simulink model "fifio_with_D2"  (R2024a)
settings: Solver=VariableStepAuto  StartTime=0.0  StopTime=0.5  RelTol=1e-3
values from neighbouring files (symbols this model uses):
  enable_FIFO_out = Ts*9009    (= 0.0675681756818)    [new_generation_coeff.m]
  Ts = 1/Fs    (= 7.50007500075e-06)    [new_generation_coeff.m]    (also in simon_test.m; simple_fft_test.m = 1/F; testPSD_c2d.m; testPSD_simulink.m)
undefined symbols (not defined in the file or in its folder): magnitude
libraries: hdlsllib x127, dsphdlxfrm2 x1
settings Model: DataTypeOverride=Off  Creator=Simon  LastModifiedBy=Simon
settings OptimizationCC: BlockReduction=off  ConditionallyExecuteInputs=off  DefaultParameterBehavior=Inlined  InheritOutputTypeSmallerThanSingle=on
settings DebuggingCC: AlgebraicLoopMsg=error  SingleTaskRateTransMsg=error  UnconnectedInputMsg=warning  UnconnectedOutputMsg=warning  UnconnectedLineMsg=warning
settings HardwareCC: ProdBitPerPointer=32  ProdBitPerSizeT=32  ProdBitPerPtrDiffT=32  ProdLargestAtomicFloat=None  ProdIntDivRoundTo=Undefined  ProdEndianess=Unspecified  ProdWordSize=32  ProdHWDeviceType=ASIC/FPGA->ASIC/FPGA  TargetBitPerPointer=64  TargetBitPerSizeT=64  TargetBitPerPtrDiffT=64  TargetLongLongMode=on  TargetIntDivRoundTo=Zero  TargetEndianess=LittleEndian  TargetWordSize=64  TargetHWDeviceType=Custom Processor->MATLAB Host Computer  ProdEqTarget=off

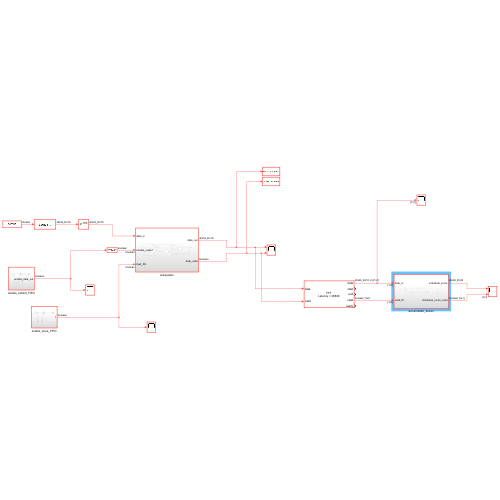
[thumbnail: Simulink's stored preview of the top-level diagram]
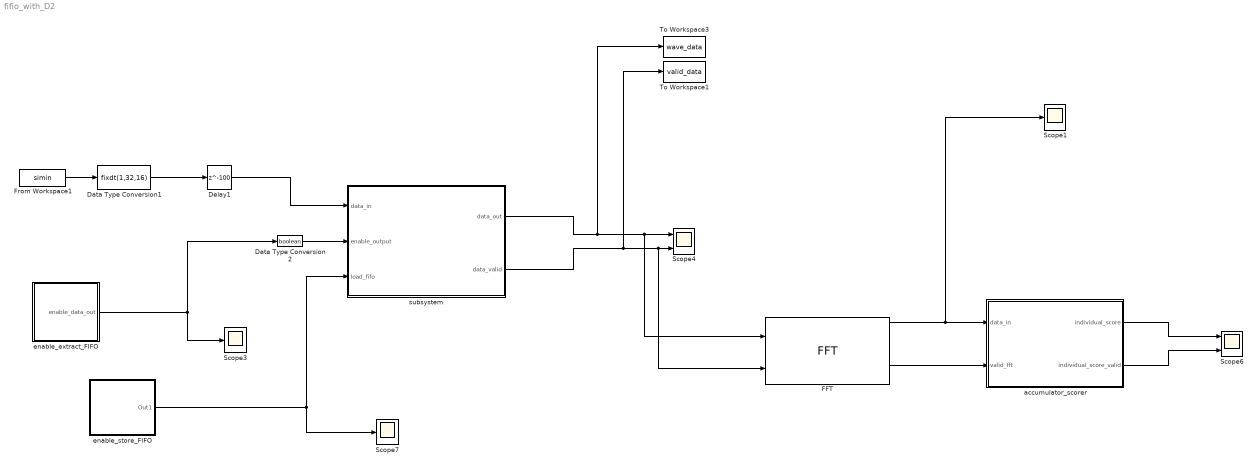
== system fifio_with_D2 ==
  Data Type Conversion1 : DataTypeConversion  OutDataTypeStr=fixdt(1,32,16)  SaturateOnIntegerOverflow=off  RndMeth=Floor
  Data Type Conversion2 : DataTypeConversion  OutDataTypeStr=boolean  SaturateOnIntegerOverflow=off  RndMeth=Floor
  Delay1 : Delay  DelayLength=100  InitialCondition=0  SampleTime=Ts
  FFT : dsphdlxfrm2/FFT  Architecture=Burst Radix 2  FFTLengthSource=Property  FFTLength=4096  FFTLengthMax=1024  ComplexMultiplication=Use 4 multipliers and 2 adders  BitReversedOutput=off  BitReversedInput=off  Normalize=off  SimulateUsing=Code generation  RoundingMethod=Floor  ResetInputPort=off  StartOutputPort=on  EndOutputPort=on
  From Workspace1 : FromWorkspace  VariableName=simin  SampleTime=Ts
  Scope1 : Scope
  Scope3 : Scope
  Scope4 : Scope  NumInputPorts=2
  Scope6 : Scope  NumInputPorts=2
  Scope7 : Scope
  To Workspace1 : ToWorkspace  VariableName=valid_data  SampleTime=Ts
  To Workspace3 : ToWorkspace  VariableName=wave_data  SampleTime=Ts
  accumulator_scorer : Subsystem
  enable_extract_FIFO : Subsystem
  enable_store_FIFO : Subsystem
  subsystem : Subsystem
  wires:
  enable_store_FIFO/1(Out1) -> subsystem/3(load_fifo), Scope7/1
  FFT/1 -> Scope1/1, accumulator_scorer/1(data_in)
  enable_extract_FIFO/1(enable_data_out) -> Data Type Conversion2/1, Scope3/1
  Data Type Conversion2/1 -> subsystem/2(enable_output)
  FFT/4 -> accumulator_scorer/2(valid_fft)
  accumulator_scorer/1(individual_score) -> Scope6/1
  Data Type Conversion1/1 -> Delay1/1
  subsystem/2(data_valid) -> FFT/2, Scope4/2, To Workspace1/1
  accumulator_scorer/2(individual_score_valid) -> Scope6/2
  From Workspace1/1 -> Data Type Conversion1/1
  Delay1/1 -> subsystem/1(data_in)
  subsystem/1(data_out) -> To Workspace3/1, FFT/1, Scope4/1

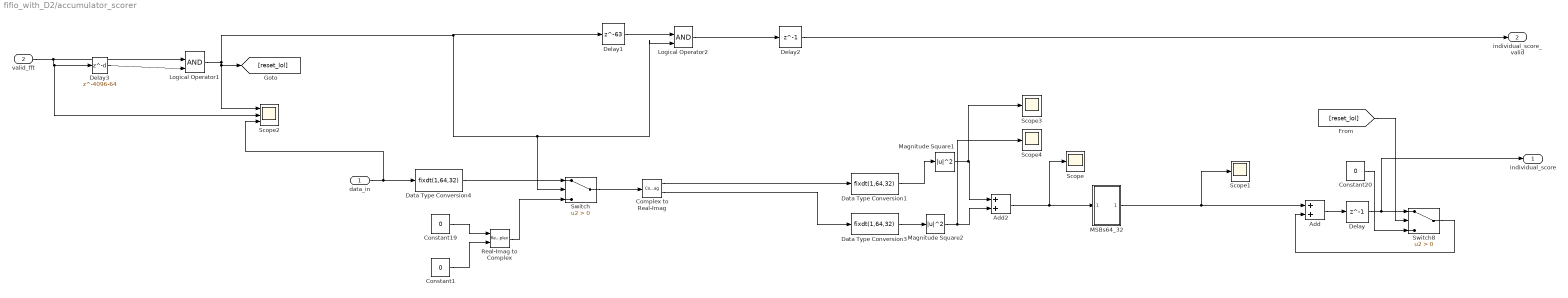
== system fifio_with_D2/accumulator_scorer ==
  data_in : Inport
  valid_fft : Inport  Port=2
  Add : Sum  OutDataTypeStr=fixdt(1,64,32)  AccumDataTypeStr=fixdt(1,64,32)
  Add2 : Sum  OutDataTypeStr=fixdt(1,64,32)  AccumDataTypeStr=fixdt(1,64,32)
  Complex to Real-Imag : ComplexToRealImag
  Constant1 : Constant  Value=0  OutDataTypeStr=fixdt(1,64,32)  SampleTime=Ts
  Constant19 : Constant  Value=0  OutDataTypeStr=fixdt(1,64,32)  SampleTime=Ts
  Constant20 : Constant  Value=0  OutDataTypeStr=fixdt(1,64,32)  SampleTime=Ts
  Data Type Conversion1 : DataTypeConversion  OutDataTypeStr=fixdt(1,64,32)  SaturateOnIntegerOverflow=off  RndMeth=Floor
  Data Type Conversion3 : DataTypeConversion  OutDataTypeStr=fixdt(1,64,32)  SaturateOnIntegerOverflow=off  RndMeth=Floor
  Data Type Conversion4 : DataTypeConversion  OutDataTypeStr=fixdt(1,64,32)  SaturateOnIntegerOverflow=off  RndMeth=Floor
  Delay : Delay  DelayLength=1  InitialCondition=0  SampleTime=Ts
  Delay1 : Delay  DelayLength=63  InitialCondition=0
  Delay2 : Delay  DelayLength=1  InitialCondition=0
  Delay3 : Delay  DelayLength=4096-64  InitialCondition=0
  Logical Operator1 : Logic  IconShape=distinctive  AllPortsSameDT=off  OutDataTypeStr=boolean
  Logical Operator2 : Logic  IconShape=distinctive  AllPortsSameDT=off  OutDataTypeStr=boolean
  MSBs64_32 : Subsystem
  Magnitude Square1 : Math  Operator=magnitude^2  SignedPower=on  OutputSignalType=real  OutDataTypeStr=fixdt(1,64,32)  RndMeth=Zero
  Magnitude Square2 : Math  Operator=magnitude^2  SignedPower=on  OutputSignalType=real  OutDataTypeStr=fixdt(1,64,32)  RndMeth=Zero
  Real-Imag to Complex : RealImagToComplex
  Scope{,1,3..4} (4 alike) : Scope
  Scope2 : Scope  NumInputPorts=3
  Switch : Switch  Criteria=u2 > Threshold  OutDataTypeStr=fixdt(1,64,32)  SaturateOnIntegerOverflow=off  InputSameDT=off
  Switch8 : Switch  Criteria=u2 > Threshold  OutDataTypeStr=fixdt(1,64,32)  SaturateOnIntegerOverflow=off  InputSameDT=off
  individual_score : Outport
  individual_score_valid : Outport  Port=2
  wires:
  Real-Imag to Complex/1 -> Switch/3
  Switch8/1 -> Add/2
  Switch/1 -> Complex to Real-Imag/1
  Delay/1 -> individual_score/1, Switch8/1
  [reset_lol] -> Switch8/2
  Add/1 -> Delay/1
  Constant20/1 -> Switch8/3
  data_in/1 -> Scope2/3, Data Type Conversion4/1
  Data Type Conversion3/1 -> Magnitude Square2/1
  Data Type Conversion1/1 -> Magnitude Square1/1
  Magnitude Square1/1 -> Scope3/1, Add2/1
  Complex to Real-Imag/1 -> Data Type Conversion1/1
  Add2/1 -> MSBs64_32/1(In1), Scope/1
  Complex to Real-Imag/2 -> Data Type Conversion3/1
  Magnitude Square2/1 -> Scope4/1, Add2/2
  Logical Operator1/1 -> Scope2/1, [reset_lol], Logical Operator2/2, Switch/2, Delay1/1
  Data Type Conversion4/1 -> Switch/1
  Constant1/1 -> Real-Imag to Complex/2
  Constant19/1 -> Real-Imag to Complex/1
  MSBs64_32/1(out) -> Scope1/1, Add/1
  Delay1/1 -> Logical Operator2/1
  Logical Operator2/1 -> Delay2/1
  Delay2/1 -> individual_score_valid/1
  valid_fft/1 -> Scope2/2, Delay3/1, Logical Operator1/1
  Delay3/1 -> Logical Operator1/2

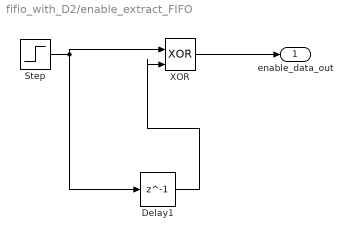
== system fifio_with_D2/enable_extract_FIFO ==
  Delay1 : Delay  DelayLength=1  InitialCondition=0  SampleTime=Ts
  Step : Step  Time=enable_FIFO_out  SampleTime=Ts
  XOR : Logic  Operator=XOR  IconShape=distinctive  AllPortsSameDT=off  OutDataTypeStr=boolean
  enable_data_out : Outport  OutDataTypeStr=boolean
  wires:
  Delay1/1 -> XOR/2
  Step/1 -> Delay1/1, XOR/1
  XOR/1 -> enable_data_out/1

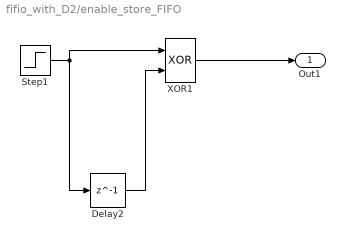
== system fifio_with_D2/enable_store_FIFO ==
  Delay2 : Delay  DelayLength=1  InitialCondition=0  SampleTime=Ts
  Step1 : Step  Time=Ts*100  SampleTime=Ts
  XOR1 : Logic  Operator=XOR  IconShape=distinctive  AllPortsSameDT=off  OutDataTypeStr=boolean
  Out1 : Outport  OutDataTypeStr=boolean
  wires:
  XOR1/1 -> Out1/1
  Step1/1 -> Delay2/1, XOR1/1
  Delay2/1 -> XOR1/2

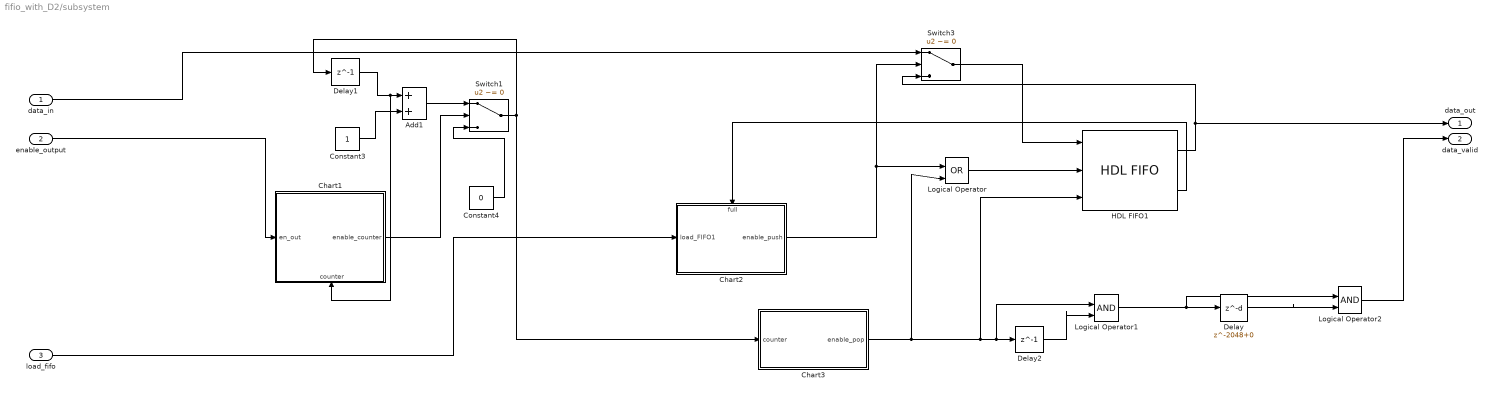
== system fifio_with_D2/subsystem ==
  data_in : Inport
  enable_output : Inport  Port=2  OutDataTypeStr=boolean
  load_fifo : Inport  Port=3  OutDataTypeStr=boolean
  Add1 : Sum  OutDataTypeStr=fixdt(0,13,0)
  Chart1 : Stateflow chart  TreatAsAtomicUnit=on
      settings: PortSchema="{\"entries\":[{\"content\":{\"sides\":[{\"content\":{\"connectorIds\":[\"In2\"]},\"type\":\"ConnectorPlacement.EquallySpacedRectSide\",\"uuid\":\"9d6f18ef-7bce-40b0-94a2-758e33355834\"},{\"content\":{\"connectorIds\":[\"Out1\"],\"side\":\"RIGHT\"},\"type\":\"ConnectorPlacement.EquallySpacedRectSide\",\"uuid\":\"7bab70ba-8111-4145-9c29-33f98ce79820\"},{\"content\":{\"side\":\"TOP\"},\"type\":\"ConnectorPlacement.EquallySpacedRectSide\",\"uuid\":\"d3288235-814f-4c71-bec2-04d07c53d63c\"},{\"content\":{\"connectorIds\":[\"In1\"],\"side\":\"BOTTOM\"},\"type\":\"ConnectorPlacement.EquallySpacedRectSide\",\"uuid\":\"018953e5-55f4-4114-8f5d-132f3f7565f7\"}]},\"type\":\"ConnectorPlacement.EquallySpacedConnector\",\"uuid\":\"70011da9-c6ae-4e69-953f-1d8cbe8c7c12\"}],\"packageUris\":[\"http://schema.mathworks.com/mf0/Connector/R2020b\"],\"version\":\"1.0\"}"
  Chart2 : Stateflow chart  TreatAsAtomicUnit=on
      settings: PortSchema="{\"entries\":[{\"content\":{\"sides\":[{\"content\":{\"connectorIds\":[\"In1\"]},\"type\":\"ConnectorPlacement.EquallySpacedRectSide\",\"uuid\":\"9d6f18ef-7bce-40b0-94a2-758e33355834\"},{\"content\":{\"connectorIds\":[\"Out1\"],\"side\":\"RIGHT\"},\"type\":\"ConnectorPlacement.EquallySpacedRectSide\",\"uuid\":\"7bab70ba-8111-4145-9c29-33f98ce79820\"},{\"content\":{\"connectorIds\":[\"In2\"],\"side\":\"TOP\"},\"type\":\"ConnectorPlacement.EquallySpacedRectSide\",\"uuid\":\"d3288235-814f-4c71-bec2-04d07c53d63c\"}]},\"type\":\"ConnectorPlacement.EquallySpacedConnector\",\"uuid\":\"70011da9-c6ae-4e69-953f-1d8cbe8c7c12\"}],\"packageUris\":[\"http://schema.mathworks.com/mf0/Connector/R2020b\"],\"version\":\"1.0\"}"
  Chart3 : Stateflow chart  TreatAsAtomicUnit=on
  Constant3 : Constant  OutDataTypeStr=fixdt(0,12,0)  SampleTime=Ts
  Constant4 : Constant  Value=0  OutDataTypeStr=fixdt(1,13,0)  SampleTime=Ts
  Delay : Delay  DelayLength=2048+0  InitialCondition=0
  Delay1 : Delay  DelayLength=1  InitialCondition=0  SampleTime=Ts
  Delay2 : Delay  DelayLength=1  InitialCondition=0  SampleTime=Ts
  HDL FIFO1 : hdlsllib/HDL RAMs/HDL FIFO  fifo_size=4096+2048+1  mode=Classic  ratio=1  push_msg=Warning  pop_msg=Warning  show_empty=off  show_full=on  show_num=off  LabelModeActiveChoice_Mode=Classic  rst_port=off
  Logical Operator : Logic  Operator=OR  IconShape=distinctive  AllPortsSameDT=off  OutDataTypeStr=boolean
  Logical Operator1 : Logic  IconShape=distinctive  AllPortsSameDT=off  OutDataTypeStr=boolean
  Logical Operator2 : Logic  IconShape=distinctive  AllPortsSameDT=off  OutDataTypeStr=boolean
  Switch1 : Switch  Criteria=u2 ~= 0  OutDataTypeStr=fixdt(0,13,0)  SaturateOnIntegerOverflow=off  InputSameDT=off
  Switch3 : Switch  Criteria=u2 ~= 0  SaturateOnIntegerOverflow=off  InputSameDT=off  OutDataTypeStr=Inherit: Same as first input
  data_out : Outport
  data_valid : Outport  Port=2
  wires:
  Delay1/1 -> Chart1/1(counter), Add1/1
  Logical Operator/1 -> HDL FIFO1/2
  HDL FIFO1/1 -> data_out/1, Switch3/3
  Switch1/1 -> Chart3/1(counter), Delay1/1
  Delay2/1 -> Logical Operator1/2
  enable_output/1 -> Chart1/2(en_out)
  Add1/1 -> Switch1/1
  Constant3/1 -> Add1/2
  HDL FIFO1/2 -> Chart2/2(full)
  Switch3/1 -> HDL FIFO1/1
  Constant4/1 -> Switch1/3
  Logical Operator1/1 -> Logical Operator2/1, Delay/1
  load_fifo/1 -> Chart2/1(load_FIFO1)
  data_in/1 -> Switch3/1
  Chart3/1(enable_pop) -> HDL FIFO1/3, Logical Operator1/1, Delay2/1, Logical Operator/2
  Chart1/1(enable_counter) -> Switch1/2
  Chart2/1(enable_push) -> Switch3/2, Logical Operator/1
  Delay/1 -> Logical Operator2/2
  Logical Operator2/1 -> data_valid/1

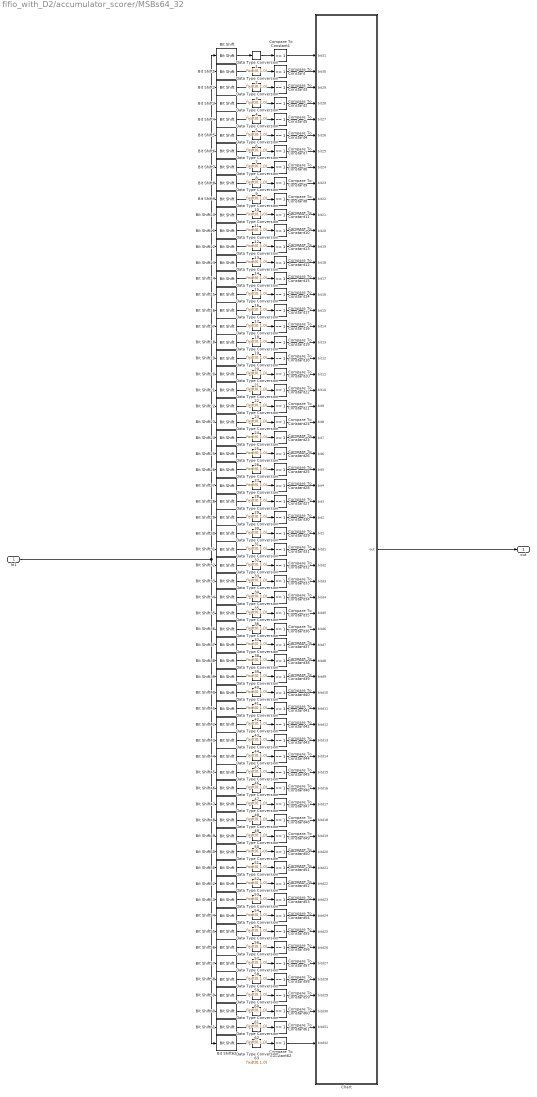
== system fifio_with_D2/accumulator_scorer/MSBs64_32 ==
  In1 : Inport
  Bit Shift : hdlsllib/Logic and Bit Operations/Bit Shift  mode=Shift Right Logical  N=30
  Bit Shift1 : hdlsllib/Logic and Bit Operations/Bit Shift  mode=Shift Right Logical  N=29
  Bit Shift10 : hdlsllib/Logic and Bit Operations/Bit Shift  mode=Shift Right Logical  N=20
  Bit Shift11 : hdlsllib/Logic and Bit Operations/Bit Shift  mode=Shift Right Logical  N=19
  Bit Shift12 : hdlsllib/Logic and Bit Operations/Bit Shift  mode=Shift Right Logical  N=18
  Bit Shift13 : hdlsllib/Logic and Bit Operations/Bit Shift  mode=Shift Right Logical  N=17
  Bit Shift14 : hdlsllib/Logic and Bit Operations/Bit Shift  mode=Shift Right Logical  N=16
  Bit Shift15 : hdlsllib/Logic and Bit Operations/Bit Shift  mode=Shift Right Logical  N=15
  Bit Shift16 : hdlsllib/Logic and Bit Operations/Bit Shift  mode=Shift Right Logical  N=14
  Bit Shift17 : hdlsllib/Logic and Bit Operations/Bit Shift  mode=Shift Right Logical  N=13
  Bit Shift18 : hdlsllib/Logic and Bit Operations/Bit Shift  mode=Shift Right Logical  N=12
  Bit Shift19 : hdlsllib/Logic and Bit Operations/Bit Shift  mode=Shift Right Logical  N=11
  Bit Shift2 : hdlsllib/Logic and Bit Operations/Bit Shift  mode=Shift Right Logical  N=28
  Bit Shift20 : hdlsllib/Logic and Bit Operations/Bit Shift  mode=Shift Right Logical  N=10
  Bit Shift21 : hdlsllib/Logic and Bit Operations/Bit Shift  mode=Shift Right Logical  N=9
  Bit Shift22 : hdlsllib/Logic and Bit Operations/Bit Shift  mode=Shift Right Logical  N=8
  Bit Shift23 : hdlsllib/Logic and Bit Operations/Bit Shift  mode=Shift Right Logical  N=7
  Bit Shift24 : hdlsllib/Logic and Bit Operations/Bit Shift  mode=Shift Right Logical  N=6
  Bit Shift25 : hdlsllib/Logic and Bit Operations/Bit Shift  mode=Shift Right Logical  N=5
  Bit Shift26 : hdlsllib/Logic and Bit Operations/Bit Shift  mode=Shift Right Logical  N=4
  Bit Shift27 : hdlsllib/Logic and Bit Operations/Bit Shift  mode=Shift Right Logical  N=3
  Bit Shift28 : hdlsllib/Logic and Bit Operations/Bit Shift  mode=Shift Right Logical  N=2
  Bit Shift29 : hdlsllib/Logic and Bit Operations/Bit Shift  mode=Shift Right Logical  N=1
  Bit Shift3 : hdlsllib/Logic and Bit Operations/Bit Shift  mode=Shift Right Logical  N=27
  Bit Shift30 : hdlsllib/Logic and Bit Operations/Bit Shift  mode=Shift Right Logical  N=0
  Bit Shift31 : hdlsllib/Logic and Bit Operations/Bit Shift  mode=Shift Left Logical  N=1
  Bit Shift32 : hdlsllib/Logic and Bit Operations/Bit Shift  mode=Shift Left Logical  N=2
  Bit Shift33 : hdlsllib/Logic and Bit Operations/Bit Shift  mode=Shift Left Logical  N=3
  Bit Shift34 : hdlsllib/Logic and Bit Operations/Bit Shift  mode=Shift Left Logical  N=4
  Bit Shift35 : hdlsllib/Logic and Bit Operations/Bit Shift  mode=Shift Left Logical  N=5
  Bit Shift36 : hdlsllib/Logic and Bit Operations/Bit Shift  mode=Shift Left Logical  N=6
  Bit Shift37 : hdlsllib/Logic and Bit Operations/Bit Shift  mode=Shift Left Logical  N=7
  Bit Shift38 : hdlsllib/Logic and Bit Operations/Bit Shift  mode=Shift Left Logical  N=8
  Bit Shift39 : hdlsllib/Logic and Bit Operations/Bit Shift  mode=Shift Left Logical  N=9
  Bit Shift4 : hdlsllib/Logic and Bit Operations/Bit Shift  mode=Shift Right Logical  N=26
  Bit Shift40 : hdlsllib/Logic and Bit Operations/Bit Shift  mode=Shift Left Logical  N=10
  Bit Shift41 : hdlsllib/Logic and Bit Operations/Bit Shift  mode=Shift Left Logical  N=11
  Bit Shift42 : hdlsllib/Logic and Bit Operations/Bit Shift  mode=Shift Left Logical  N=12
  Bit Shift43 : hdlsllib/Logic and Bit Operations/Bit Shift  mode=Shift Left Logical  N=13
  Bit Shift44 : hdlsllib/Logic and Bit Operations/Bit Shift  mode=Shift Left Logical  N=14
  Bit Shift45 : hdlsllib/Logic and Bit Operations/Bit Shift  mode=Shift Left Logical  N=15
  Bit Shift46 : hdlsllib/Logic and Bit Operations/Bit Shift  mode=Shift Left Logical  N=16
  Bit Shift47 : hdlsllib/Logic and Bit Operations/Bit Shift  mode=Shift Left Logical  N=17
  Bit Shift48 : hdlsllib/Logic and Bit Operations/Bit Shift  mode=Shift Left Logical  N=18
  Bit Shift49 : hdlsllib/Logic and Bit Operations/Bit Shift  mode=Shift Left Logical  N=19
  Bit Shift5 : hdlsllib/Logic and Bit Operations/Bit Shift  mode=Shift Right Logical  N=25
  Bit Shift50 : hdlsllib/Logic and Bit Operations/Bit Shift  mode=Shift Left Logical  N=20
  Bit Shift51 : hdlsllib/Logic and Bit Operations/Bit Shift  mode=Shift Left Logical  N=21
  Bit Shift52 : hdlsllib/Logic and Bit Operations/Bit Shift  mode=Shift Left Logical  N=22
  Bit Shift53 : hdlsllib/Logic and Bit Operations/Bit Shift  mode=Shift Left Logical  N=23
  Bit Shift54 : hdlsllib/Logic and Bit Operations/Bit Shift  mode=Shift Left Logical  N=24
  Bit Shift55 : hdlsllib/Logic and Bit Operations/Bit Shift  mode=Shift Left Logical  N=25
  Bit Shift56 : hdlsllib/Logic and Bit Operations/Bit Shift  mode=Shift Left Logical  N=26
  Bit Shift57 : hdlsllib/Logic and Bit Operations/Bit Shift  mode=Shift Left Logical  N=27
  Bit Shift58 : hdlsllib/Logic and Bit Operations/Bit Shift  mode=Shift Left Logical  N=28
  Bit Shift59 : hdlsllib/Logic and Bit Operations/Bit Shift  mode=Shift Left Logical  N=29
  Bit Shift6 : hdlsllib/Logic and Bit Operations/Bit Shift  mode=Shift Right Logical  N=24
  Bit Shift60 : hdlsllib/Logic and Bit Operations/Bit Shift  mode=Shift Left Logical  N=30
  Bit Shift61 : hdlsllib/Logic and Bit Operations/Bit Shift  mode=Shift Left Logical  N=31
  Bit Shift62 : hdlsllib/Logic and Bit Operations/Bit Shift  mode=Shift Left Logical  N=32
  Bit Shift7 : hdlsllib/Logic and Bit Operations/Bit Shift  mode=Shift Right Logical  N=23
  Bit Shift8 : hdlsllib/Logic and Bit Operations/Bit Shift  mode=Shift Right Logical  N=22
  Bit Shift9 : hdlsllib/Logic and Bit Operations/Bit Shift  mode=Shift Right Logical  N=21
  Chart : Stateflow chart  TreatAsAtomicUnit=on
  Compare To Constant{,1..62} (63 alike) : hdlsllib/Logic and Bit Operations/Compare To Constant  relop===  const=1  OutDataTypeStr=boolean
  Data Type Conversion{1..63} (63 alike) : DataTypeConversion  OutDataTypeStr=fixdt(0,1,0)  SaturateOnIntegerOverflow=off  RndMeth=Floor
  out : Outport
  wires:
  Bit Shift/1 -> Data Type Conversion1/1
  Chart/1(out) -> out/1
  In1/1 -> Bit Shift/1, Bit Shift1/1, Bit Shift2/1, Bit Shift3/1, Bit Shift4/1, Bit Shift5/1, Bit Shift6/1, Bit Shift7/1, Bit Shift8/1, Bit Shift9/1, Bit Shift10/1, Bit Shift11/1, Bit Shift12/1, Bit Shift13/1, Bit Shift14/1, Bit Shift15/1, Bit Shift16/1, Bit Shift17/1, Bit Shift18/1, Bit Shift19/1, Bit Shift20/1, Bit Shift21/1, Bit Shift22/1, Bit Shift23/1, Bit Shift24/1, Bit Shift25/1, Bit Shift26/1, Bit Shift27/1, Bit Shift28/1, Bit Shift29/1, Bit Shift30/1, Bit Shift31/1, Bit Shift62/1, Bit Shift61/1, Bit Shift60/1, Bit Shift59/1, Bit Shift58/1, Bit Shift57/1, Bit Shift56/1, Bit Shift55/1, Bit Shift54/1, Bit Shift53/1, Bit Shift52/1, Bit Shift51/1, Bit Shift50/1, Bit Shift49/1, Bit Shift48/1, Bit Shift47/1, Bit Shift46/1, Bit Shift45/1, Bit Shift44/1, Bit Shift43/1, Bit Shift42/1, Bit Shift41/1, Bit Shift40/1, Bit Shift39/1, Bit Shift38/1, Bit Shift37/1, Bit Shift36/1, Bit Shift35/1, Bit Shift34/1, Bit Shift33/1, Bit Shift32/1
  Data Type Conversion1/1 -> Compare To Constant1/1
  Data Type Conversion2/1 -> Compare To Constant/1
  Bit Shift1/1 -> Data Type Conversion2/1
  Bit Shift2/1 -> Data Type Conversion3/1
  Data Type Conversion3/1 -> Compare To Constant3/1
  Data Type Conversion4/1 -> Compare To Constant2/1
  Bit Shift3/1 -> Data Type Conversion4/1
  Bit Shift4/1 -> Data Type Conversion5/1
  Data Type Conversion5/1 -> Compare To Constant5/1
  Bit Shift6/1 -> Data Type Conversion7/1
  Data Type Conversion7/1 -> Compare To Constant7/1
  Data Type Conversion6/1 -> Compare To Constant4/1
  Bit Shift5/1 -> Data Type Conversion6/1
  Data Type Conversion9/1 -> Compare To Constant9/1
  Bit Shift7/1 -> Data Type Conversion8/1
  Bit Shift12/1 -> Data Type Conversion13/1
  Bit Shift11/1 -> Data Type Conversion12/1
  Data Type Conversion13/1 -> Compare To Constant13/1
  Data Type Conversion8/1 -> Compare To Constant6/1
  Data Type Conversion11/1 -> Compare To Constant11/1
  Bit Shift9/1 -> Data Type Conversion10/1
  Bit Shift10/1 -> Data Type Conversion11/1
  Data Type Conversion10/1 -> Compare To Constant8/1
  Data Type Conversion12/1 -> Compare To Constant10/1
  Bit Shift8/1 -> Data Type Conversion9/1
  Data Type Conversion15/1 -> Compare To Constant15/1
  Bit Shift13/1 -> Data Type Conversion14/1
  Bit Shift18/1 -> Data Type Conversion19/1
  Bit Shift17/1 -> Data Type Conversion18/1
  Data Type Conversion19/1 -> Compare To Constant19/1
  Data Type Conversion14/1 -> Compare To Constant12/1
  Data Type Conversion17/1 -> Compare To Constant17/1
  Bit Shift15/1 -> Data Type Conversion16/1
  Bit Shift16/1 -> Data Type Conversion17/1
  Data Type Conversion16/1 -> Compare To Constant14/1
  Data Type Conversion18/1 -> Compare To Constant16/1
  Bit Shift14/1 -> Data Type Conversion15/1
  Data Type Conversion21/1 -> Compare To Constant20/1
  Bit Shift19/1 -> Data Type Conversion20/1
  Bit Shift24/1 -> Data Type Conversion25/1
  Bit Shift23/1 -> Data Type Conversion24/1
  Data Type Conversion25/1 -> Compare To Constant23/1
  Data Type Conversion20/1 -> Compare To Constant18/1
  Data Type Conversion23/1 -> Compare To Constant21/1
  Bit Shift21/1 -> Data Type Conversion22/1
  Bit Shift22/1 -> Data Type Conversion23/1
  Data Type Conversion22/1 -> Compare To Constant22/1
  Data Type Conversion24/1 -> Compare To Constant24/1
  Bit Shift20/1 -> Data Type Conversion21/1
  Data Type Conversion27/1 -> Compare To Constant25/1
  Bit Shift25/1 -> Data Type Conversion26/1
  Bit Shift30/1 -> Data Type Conversion31/1
  Bit Shift29/1 -> Data Type Conversion30/1
  Data Type Conversion31/1 -> Compare To Constant29/1
  Data Type Conversion26/1 -> Compare To Constant26/1
  Data Type Conversion29/1 -> Compare To Constant27/1
  Bit Shift27/1 -> Data Type Conversion28/1
  Bit Shift28/1 -> Data Type Conversion29/1
  Data Type Conversion28/1 -> Compare To Constant28/1
  Data Type Conversion30/1 -> Compare To Constant30/1
  Bit Shift26/1 -> Data Type Conversion27/1
  Bit Shift31/1 -> Data Type Conversion32/1
  Data Type Conversion32/1 -> Compare To Constant31/1
  Data Type Conversion33/1 -> Compare To Constant32/1
  Bit Shift32/1 -> Data Type Conversion33/1
  Data Type Conversion34/1 -> Compare To Constant33/1
  Bit Shift33/1 -> Data Type Conversion34/1
  Data Type Conversion35/1 -> Compare To Constant34/1
  Bit Shift34/1 -> Data Type Conversion35/1
  Data Type Conversion36/1 -> Compare To Constant35/1
  Bit Shift35/1 -> Data Type Conversion36/1
  Data Type Conversion37/1 -> Compare To Constant36/1
  Bit Shift36/1 -> Data Type Conversion37/1
  Data Type Conversion39/1 -> Compare To Constant38/1
  Data Type Conversion43/1 -> Compare To Constant42/1
  Bit Shift41/1 -> Data Type Conversion42/1
  Data Type Conversion42/1 -> Compare To Constant41/1
  Bit Shift42/1 -> Data Type Conversion43/1
  Data Type Conversion41/1 -> Compare To Constant40/1
  Bit Shift40/1 -> Data Type Conversion41/1
  Bit Shift39/1 -> Data Type Conversion40/1
  Data Type Conversion38/1 -> Compare To Constant37/1
  Data Type Conversion40/1 -> Compare To Constant39/1
  Bit Shift38/1 -> Data Type Conversion39/1
  Bit Shift37/1 -> Data Type Conversion38/1
  Data Type Conversion45/1 -> Compare To Constant44/1
  Data Type Conversion49/1 -> Compare To Constant48/1
  Bit Shift47/1 -> Data Type Conversion48/1
  Data Type Conversion48/1 -> Compare To Constant47/1
  Bit Shift48/1 -> Data Type Conversion49/1
  Data Type Conversion47/1 -> Compare To Constant46/1
  Bit Shift46/1 -> Data Type Conversion47/1
  Bit Shift45/1 -> Data Type Conversion46/1
  Data Type Conversion44/1 -> Compare To Constant43/1
  Data Type Conversion46/1 -> Compare To Constant45/1
  Bit Shift44/1 -> Data Type Conversion45/1
  Bit Shift43/1 -> Data Type Conversion44/1
  Data Type Conversion51/1 -> Compare To Constant50/1
  Data Type Conversion55/1 -> Compare To Constant54/1
  Bit Shift53/1 -> Data Type Conversion54/1
  Data Type Conversion54/1 -> Compare To Constant53/1
  Bit Shift54/1 -> Data Type Conversion55/1
  Data Type Conversion53/1 -> Compare To Constant52/1
  Bit Shift52/1 -> Data Type Conversion53/1
  Bit Shift51/1 -> Data Type Conversion52/1
  Data Type Conversion50/1 -> Compare To Constant49/1
  Data Type Conversion52/1 -> Compare To Constant51/1
  Bit Shift50/1 -> Data Type Conversion51/1
  Bit Shift49/1 -> Data Type Conversion50/1
  Data Type Conversion57/1 -> Compare To Constant56/1
  Data Type Conversion61/1 -> Compare To Constant60/1
  Bit Shift59/1 -> Data Type Conversion60/1
  Data Type Conversion60/1 -> Compare To Constant59/1
  Bit Shift60/1 -> Data Type Conversion61/1
  Data Type Conversion59/1 -> Compare To Constant58/1
  Bit Shift58/1 -> Data Type Conversion59/1
  Bit Shift57/1 -> Data Type Conversion58/1
  Data Type Conversion56/1 -> Compare To Constant55/1
  Data Type Conversion58/1 -> Compare To Constant57/1
  Bit Shift56/1 -> Data Type Conversion57/1
  Bit Shift55/1 -> Data Type Conversion56/1
  Bit Shift61/1 -> Data Type Conversion62/1
  Data Type Conversion62/1 -> Compare To Constant61/1
  Data Type Conversion63/1 -> Compare To Constant62/1
  Bit Shift62/1 -> Data Type Conversion63/1
  Compare To Constant1/1 -> Chart/1(bit31)
  Compare To Constant/1 -> Chart/2(bit30)
  Compare To Constant3/1 -> Chart/3(bit29)
  Compare To Constant2/1 -> Chart/4(bit28)
  Compare To Constant5/1 -> Chart/5(bit27)
  Compare To Constant4/1 -> Chart/6(bit26)
  Compare To Constant7/1 -> Chart/7(bit25)
  Compare To Constant6/1 -> Chart/8(bit24)
  Compare To Constant9/1 -> Chart/9(bit23)
  Compare To Constant8/1 -> Chart/10(bit22)
  Compare To Constant11/1 -> Chart/11(bit21)
  Compare To Constant10/1 -> Chart/12(bit20)
  Compare To Constant13/1 -> Chart/13(bit19)
  Compare To Constant12/1 -> Chart/14(bit18)
  Compare To Constant15/1 -> Chart/15(bit17)
  Compare To Constant14/1 -> Chart/16(bit16)
  Compare To Constant17/1 -> Chart/17(bit15)
  Compare To Constant16/1 -> Chart/18(bit14)
  Compare To Constant19/1 -> Chart/19(bit13)
  Compare To Constant18/1 -> Chart/20(bit12)
  Compare To Constant20/1 -> Chart/21(bit11)
  Compare To Constant22/1 -> Chart/22(bit10)
  Compare To Constant21/1 -> Chart/23(bit9)
  Compare To Constant24/1 -> Chart/24(bit8)
  Compare To Constant23/1 -> Chart/25(bit7)
  Compare To Constant26/1 -> Chart/26(bit6)
  Compare To Constant25/1 -> Chart/27(bit5)
  Compare To Constant28/1 -> Chart/28(bit4)
  Compare To Constant27/1 -> Chart/29(bit3)
  Compare To Constant30/1 -> Chart/30(bit2)
  Compare To Constant29/1 -> Chart/31(bit1)
  Compare To Constant31/1 -> Chart/32(bitd1)
  Compare To Constant32/1 -> Chart/33(bitd2)
  Compare To Constant33/1 -> Chart/34(bitd3)
  Compare To Constant34/1 -> Chart/35(bitd4)
  Compare To Constant35/1 -> Chart/36(bitd5)
  Compare To Constant36/1 -> Chart/37(bitd6)
  Compare To Constant37/1 -> Chart/38(bitd7)
  Compare To Constant38/1 -> Chart/39(bitd8)
  Compare To Constant39/1 -> Chart/40(bitd9)
  Compare To Constant40/1 -> Chart/41(bitd10)
  Compare To Constant41/1 -> Chart/42(bitd11)
  Compare To Constant42/1 -> Chart/43(bitd12)
  Compare To Constant43/1 -> Chart/44(bitd13)
  Compare To Constant44/1 -> Chart/45(bitd14)
  Compare To Constant45/1 -> Chart/46(bitd15)
  Compare To Constant46/1 -> Chart/47(bitd16)
  Compare To Constant47/1 -> Chart/48(bitd17)
  Compare To Constant48/1 -> Chart/49(bitd18)
  Compare To Constant49/1 -> Chart/50(bitd19)
  Compare To Constant50/1 -> Chart/51(bitd20)
  Compare To Constant51/1 -> Chart/52(bitd21)
  Compare To Constant52/1 -> Chart/53(bitd22)
  Compare To Constant53/1 -> Chart/54(bitd23)
  Compare To Constant54/1 -> Chart/55(bitd24)
  Compare To Constant55/1 -> Chart/56(bitd25)
  Compare To Constant56/1 -> Chart/57(bitd26)
  Compare To Constant57/1 -> Chart/58(bitd27)
  Compare To Constant58/1 -> Chart/59(bitd28)
  Compare To Constant59/1 -> Chart/60(bitd29)
  Compare To Constant60/1 -> Chart/61(bitd30)
  Compare To Constant61/1 -> Chart/62(bitd31)
  Compare To Constant62/1 -> Chart/63(bitd32)

== stateflow chart fifio_with_D2/subsystem/Chart1 ==
  settings: updateMethod=DISCRETE  sampleTime=Ts  executeAtInitialization=1
  state initial_counter
    during:
    enable_counter = false;
  state counter_state
    during:
    enable_counter = true;
  (default) -> initial_counter
  counter_state -> initial_counter : [counter == 1+(4096+2048+1)]
  initial_counter -> counter_state : [en_out == true]
  data: counter input fixdt(0,13,0); enable_counter output boolean; en_out input boolean

== stateflow chart fifio_with_D2/subsystem/Chart2 ==
  settings: updateMethod=DISCRETE  sampleTime=Ts  executeAtInitialization=1
  state initial_push
    during:
    enable_push = false;
  state push_state
    during:
    enable_push = true;
  (default) -> initial_push
  push_state -> initial_push : [full == true]
  initial_push -> push_state : [load_FIFO1 == true]
  data: load_FIFO1 input boolean; full input boolean; enable_push output boolean

== stateflow chart fifio_with_D2/accumulator_scorer/MSBs64_32/Chart ==
  settings: executeAtInitialization=1
  state state_lol
    during:
    out = 0;
  state MSBout
    entry:
    out = 30;
  state MSBout1
    entry:
    out = 29;
  state MSBout2
    entry:
    out = 28;
  state MSBout3
    entry:
    out = 27;
  state MSBout5
    entry:
    out = 26;
  state MSBout7
    entry:
    out = 25;
  state MSBout4
    entry:
    out = 24;
  state MSBout6
    entry:
    out = 23;
  state MSBout13
    entry:
    out = 22;
  state MSBout15
    entry:
    out = 21;
  state MSBout12
    entry:
    out = 20;
  state MSBout14
    entry:
    out = 19;
  state MSBout10
    entry:
    out = 18;
  state MSBout9
    entry:
    out = 17;
  state MSBout8
    entry:
    out = 16;
  state MSBout11
    entry:
    out = 15;
  state MSBout17
    entry:
    out = 14;
  state MSBout16
    entry:
    out = 13;
  state MSBout18
    entry:
    out = 12;
  state MSBout22
    entry:
    out = 11;
  state MSBout20
    entry:
    out = 10;
  state MSBout19
    entry:
    out = 9;
  state MSBout21
    entry:
    out = 8;
  state MSBout24
    entry:
    out = 7;
  state MSBout23
    entry:
    out = 6;
  state MSBout25
    entry:
    out = 5;
  state MSBout29
    entry:
    out = 4;
  state MSBout27
    entry:
    out = 3;
  state MSBout26
    entry:
    out = 2;
  state MSBout28
    entry:
    out = 1;
  state MSBout30
    entry:
    out = 0;
  state MSBout31
    entry:
    out = -1;
  state MSBout32
    entry:
    out = -2;
  state MSBout33
    entry:
    out = -3;
  state MSBout34
    entry:
    out = -4;
  state MSBout35
    entry:
    out = -5;
  state MSBout38
    entry:
    out = -6;
  state MSBout44
    entry:
    out = -7;
  state MSBout46
    entry:
    out = -8;
  state MSBout50
    entry:
    out = -9;
  state MSBout39
    entry:
    out = -10;
  state MSBout36
    entry:
    out = -11;
  state MSBout53
    entry:
    out = -12;
  state MSBout48
    entry:
    out = -13;
  state MSBout47
    entry:
    out = -14;
  state MSBout54
    entry:
    out = -15;
  state MSBout37
    entry:
    out = -16;
  state MSBout55
    entry:
    out = -17;
  state MSBout60
    entry:
    out = -18;
  state MSBout42
    entry:
    out = -19;
  state MSBout45
    entry:
    out = -20;
  state MSBout51
    entry:
    out = -21;
  state MSBout40
    entry:
    out = -22;
  state MSBout49
    entry:
    out = -23;
  state MSBout61
    entry:
    out = -24;
  state MSBout56
    entry:
    out = -25;
  state MSBout43
    entry:
    out = -26;
  state MSBout41
    entry:
    out = -27;
  state MSBout58
    entry:
    out = -28;
  state MSBout57
    entry:
    out = -29;
  state MSBout59
    entry:
    out = -30;
  state MSBout52
    entry:
    out = -31;
  state MSBout62
    entry:
    out = -32;
  (default) -> state_lol
  state_lol -> MSBout [order 1] : [bit31==true]
  MSBout -> state_lol
  state_lol -> MSBout1 [order 2] : [bit30==true]
  MSBout1 -> state_lol
  state_lol -> MSBout2 [order 3] : [bit29==true]
  MSBout2 -> state_lol
  state_lol -> MSBout3 [order 4] : [bit28==true]
  MSBout3 -> state_lol
  state_lol -> MSBout5 [order 5] : [bit27==true]
  MSBout5 -> state_lol
  state_lol -> MSBout7 [order 6] : [bit26==true]
  MSBout7 -> state_lol
  state_lol -> MSBout4 [order 7] : [bit25==true]
  MSBout4 -> state_lol
  state_lol -> MSBout6 [order 8] : [bit24==true]
  MSBout6 -> state_lol
  state_lol -> MSBout13 [order 9] : [bit23==true]
  MSBout13 -> state_lol
  state_lol -> MSBout15 [order 10] : [bit22==true]
  MSBout15 -> state_lol
  state_lol -> MSBout12 [order 11] : [bit21==true]
  MSBout12 -> state_lol
  state_lol -> MSBout14 [order 12] : [bit20==true]
  MSBout14 -> state_lol
  state_lol -> MSBout10 [order 13] : [bit19==true]
  MSBout10 -> state_lol
  state_lol -> MSBout9 [order 14] : [bit18==true]
  MSBout9 -> state_lol
  state_lol -> MSBout8 [order 15] : [bit17==true]
  MSBout8 -> state_lol
  state_lol -> MSBout11 [order 16] : [bit16==true]
  MSBout11 -> state_lol
  state_lol -> MSBout17 [order 17] : [bit15==true]
  MSBout17 -> state_lol
  state_lol -> MSBout16 [order 18] : [bit14==true]
  MSBout16 -> state_lol
  state_lol -> MSBout18 [order 19] : [bit13==true]
  MSBout18 -> state_lol
  state_lol -> MSBout22 [order 20] : [bit12==true]
  MSBout22 -> state_lol
  state_lol -> MSBout20 [order 21] : [bit11==true]
  MSBout20 -> state_lol
  state_lol -> MSBout19 [order 22] : [bit10==true]
  MSBout19 -> state_lol
  state_lol -> MSBout21 [order 23] : [bit9==true]
  MSBout21 -> state_lol
  state_lol -> MSBout24 [order 24] : [bit8==true]
  MSBout24 -> state_lol
  state_lol -> MSBout23 [order 25] : [bit7==true]
  MSBout23 -> state_lol
  state_lol -> MSBout25 [order 26] : [bit6==true]
  MSBout25 -> state_lol
  state_lol -> MSBout29 [order 27] : [bit5==true]
  MSBout29 -> state_lol
  state_lol -> MSBout27 [order 28] : [bit4==true]
  MSBout27 -> state_lol
  state_lol -> MSBout26 [order 29] : [bit3==true]
  MSBout26 -> state_lol
  state_lol -> MSBout28 [order 30] : [bit2==true]
  MSBout28 -> state_lol
  state_lol -> MSBout30 [order 31] : [bit1==true]
  MSBout30 -> state_lol
  state_lol -> MSBout31 [order 32] : [bitd1==true]
  MSBout31 -> state_lol
  state_lol -> MSBout32 [order 33] : [bitd2==true]
  MSBout32 -> state_lol
  state_lol -> MSBout33 [order 34] : [bitd3==true]
  MSBout33 -> state_lol
  state_lol -> MSBout34 [order 35] : [bitd4==true]
  MSBout34 -> state_lol
  state_lol -> MSBout35 [order 36] : [bitd5==true]
  MSBout35 -> state_lol
  state_lol -> MSBout38 [order 37] : [bitd6==true]
  MSBout38 -> state_lol
  state_lol -> MSBout44 [order 38] : [bitd7==true]
  MSBout44 -> state_lol
  state_lol -> MSBout46 [order 39] : [bitd8==true]
  MSBout46 -> state_lol
  state_lol -> MSBout50 [order 40] : [bitd9==true]
  MSBout50 -> state_lol
  state_lol -> MSBout39 [order 41] : [bitd10==true]
  MSBout39 -> state_lol
  state_lol -> MSBout36 [order 42] : [bitd11==true]
  MSBout36 -> state_lol
  state_lol -> MSBout53 [order 43] : [bitd12==true]
  MSBout53 -> state_lol
  state_lol -> MSBout48 [order 44] : [bitd13==true]
  MSBout48 -> state_lol
  state_lol -> MSBout47 [order 45] : [bitd14==true]
  MSBout47 -> state_lol
  state_lol -> MSBout54 [order 46] : [bitd15==true]
  MSBout54 -> state_lol
  state_lol -> MSBout37 [order 47] : [bitd16==true]
  MSBout37 -> state_lol
  state_lol -> MSBout55 [order 48] : [bitd17==true]
  MSBout55 -> state_lol
  state_lol -> MSBout60 [order 49] : [bitd18==true]
  MSBout60 -> state_lol
  state_lol -> MSBout42 [order 50] : [bitd19==true]
  MSBout42 -> state_lol
  state_lol -> MSBout45 [order 51] : [bitd20==true]
  MSBout45 -> state_lol
  state_lol -> MSBout51 [order 52] : [bitd21==true]
  MSBout51 -> state_lol
  state_lol -> MSBout40 [order 53] : [bitd22==true]
  MSBout40 -> state_lol
  state_lol -> MSBout49 [order 54] : [bitd23==true]
  MSBout49 -> state_lol
  state_lol -> MSBout61 [order 55] : [bitd24==true]
  MSBout61 -> state_lol
  state_lol -> MSBout56 [order 56] : [bitd25==true]
  MSBout56 -> state_lol
  state_lol -> MSBout43 [order 57] : [bitd26==true]
  MSBout43 -> state_lol
  state_lol -> MSBout41 [order 58] : [bitd27==true]
  MSBout41 -> state_lol
  state_lol -> MSBout58 [order 59] : [bitd28==true]
  MSBout58 -> state_lol
  state_lol -> MSBout57 [order 60] : [bitd29==true]
  MSBout57 -> state_lol
  state_lol -> MSBout59 [order 61] : [bitd30==true]
  MSBout59 -> state_lol
  state_lol -> MSBout52 [order 62] : [bitd31==true]
  MSBout52 -> state_lol
  state_lol -> MSBout62 [order 63] : [bitd32==true]
  MSBout62 -> state_lol
  data: bit31 input; bit30 input; bit29 input; bit28 input; bit27 input; bit26 input; bit25 input; bit24 input; bit23 input; bit22 input; bit21 input; bit20 input; bit19 input; bit18 input; bit17 input; bit16 input; bit15 input; bit14 input; bit13 input; bit12 input; bit11 input; bit10 input; bit9 input; bit8 input; bit7 input; out output fixdt(1,8,0); bit6 input; bit5 input; bit4 input; bit3 input; bit2 input; bit1 input; bitd1 input; bitd2 input; bitd3 input; bitd4 input; bitd5 input; bitd6 input; bitd7 input; bitd8 input; bitd9 input; bitd10 input; bitd11 input; bitd12 input; bitd13 input; bitd14 input; bitd15 input; bitd16 input; bitd17 input; bitd18 input; bitd19 input; bitd20 input; bitd21 input; bitd22 input; bitd23 input; bitd24 input; bitd25 input; bitd26 input; bitd27 input; bitd28 input; bitd29 input; bitd30 input; bitd31 input; bitd32 input

== stateflow chart fifio_with_D2/subsystem/Chart3 ==
  settings: updateMethod=DISCRETE  sampleTime=Ts  executeAtInitialization=1
  state initial_popstate
    during:
    enable_pop = false;
  state pop_state
    during:
    enable_pop = true;
  (default) -> initial_popstate
  pop_state -> initial_popstate : [counter == 2+(4096+2048+1)]
  initial_popstate -> pop_state : [counter == 1]
  data: enable_pop output boolean; counter input fixdt(0,13,0)
